simulink model "quadcopterfinal"  (R2015a)
settings: Solver=ode45  SolverMode=SingleTasking  StartTime=0.0  StopTime=10  MaxStep=0.02  RelTol=1e-3
InitFcn:
  | parameters
undefined symbols (not defined in the file or in its folder): kd_roll_rate, kd_yaw_rate, kd_z_rate, ki_roll_rate, ki_yaw_rate, ki_z_rate, kp_roll, kp_roll_rate, kp_yaw, kp_yaw_rate, kp_z, kp_z_rate
libraries: simulink x4
settings Model: CovMetricSettings=dwe  CovHtmlReporting=off  covSaveCumulativeToWorkspaceVar=off  CovSaveSingleToWorkspaceVar=off  CovExternalEMLEnable=on  Creator=manoj  LastModifiedBy=manoj
settings DataIOCC: LimitDataPoints=off  SaveFormat=Dataset
settings DebuggingCC: SFUnexpectedBacktrackingDiag=error  SFNoUnconditionalDefaultTransitionDiag=error
settings HardwareCC: ProdBitPerPointer=64  ProdLargestAtomicFloat=Float  ProdIntDivRoundTo=Zero  ProdEndianess=LittleEndian  ProdHWDeviceType=Specified
settings ModelReferenceCC: PropagateSignalLabelsOutOfModel=on
settings GRTTargetCC: TargetLangStandard=C99 (ISO)  GeneratePreprocessorConditionals=Use local settings

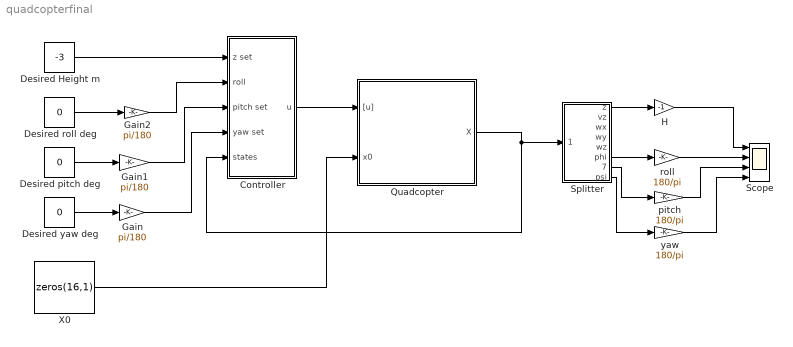
== system quadcopterfinal ==
  Controller : Subsystem
  Desired Height m : Constant  Value=-3
  Desired pitch deg : Constant  Value=0
  Desired roll deg : Constant  Value=0
  Desired yaw deg : Constant  Value=0
  Gain : Gain  Gain=pi/180
  Gain1 : Gain  Gain=pi/180
  Gain2 : Gain  Gain=pi/180
  H : Gain  Gain=-1
  Quadcopter : Subsystem
      mask Display: image('/home/manoj/gits/DDP_work/FCB related/quadcopter simulation/quad render 1(1).png');
  Scope : Scope  NumInputPorts=4
      settings: TimeRange=auto  ShowLegends=on  MaxDataPoints=5000  SaveToWorkspace=off  SaveName=ScopeData  YMin=-551.8125~-5~-5~-5  YMax=61.3125~5~5~5  SampleTime=-1
  Splitter : MATLAB Function  TreatAsAtomicUnit=on
      settings: PermitHierarchicalResolution=ParametersOnly
  X0 : Constant  Value=zeros(16,1)
  pitch : Gain  Gain=180/pi
  roll : Gain  Gain=180/pi
  yaw : Gain  Gain=180/pi
  wires:
  X0/1 -> Quadcopter/2(x0)
  Quadcopter/1(X) -> Splitter/1(states), Controller/5(states)
  Desired Height m/1 -> Controller/1(z set)
  Desired roll deg/1 -> Gain2/1
  Desired pitch deg/1 -> Gain1/1
  Desired yaw deg/1 -> Gain/1
  Controller/1(u) -> Quadcopter/1("[u]")
  Splitter/1(z) -> H/1
  Splitter/7(theta) -> pitch/1
  Splitter/8(psi) -> yaw/1
  H/1 -> Scope/1
  Gain1/1 -> Controller/3(pitch set)
  Gain/1 -> Controller/4(yaw set)
  roll/1 -> Scope/2
  pitch/1 -> Scope/3
  yaw/1 -> Scope/4
  Splitter/6(phi) -> roll/1
  Gain2/1 -> Controller/2(roll)

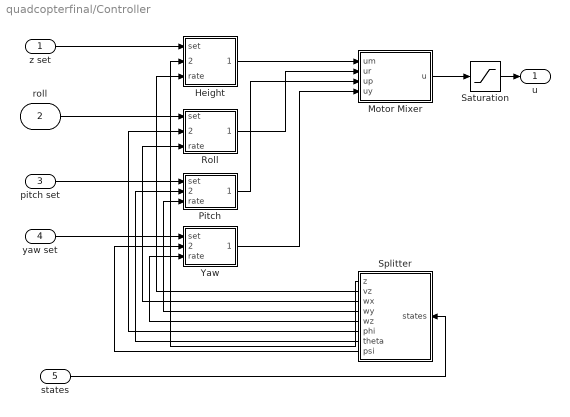
== system quadcopterfinal/Controller ==
  z set : Inport
  roll : Inport  Port=2
  pitch set : Inport  Port=3
  yaw set : Inport  Port=4
  states : Inport  Port=5
  Height : Subsystem
  Motor Mixer : MATLAB Function  TreatAsAtomicUnit=on
      settings: PermitHierarchicalResolution=ParametersOnly
  Pitch : Subsystem
  Roll : Subsystem
  Saturation : Saturate  UpperLimit=1  LowerLimit=0
  Splitter : MATLAB Function  TreatAsAtomicUnit=on
      settings: PermitHierarchicalResolution=ParametersOnly
  Yaw : Subsystem
  u : Outport
  wires:
  Splitter/3(wx) -> Roll/3(rate)
  Splitter/7(theta) -> Pitch/2(state)
  Splitter/1(z) -> Height/2(state)
  Splitter/8(psi) -> Yaw/2(state)
  Motor Mixer/1(u) -> Saturation/1
  z set/1 -> Height/1(set)
  Height/1(Out1) -> Motor Mixer/1(um)
  Roll/1(Out1) -> Motor Mixer/2(ur)
  Pitch/1(Out1) -> Motor Mixer/3(up)
  Yaw/1(Out1) -> Motor Mixer/4(uy)
  roll/1 -> Roll/1(set)
  pitch set/1 -> Pitch/1(set)
  yaw set/1 -> Yaw/1(set)
  Splitter/4(wy) -> Pitch/3(rate)
  Splitter/2(vz) -> Height/3(rate)
  Splitter/6(phi) -> Roll/2(state)
  Splitter/5(wz) -> Yaw/3(rate)
  Saturation/1 -> u/1
  states/1 -> Splitter/1(states)

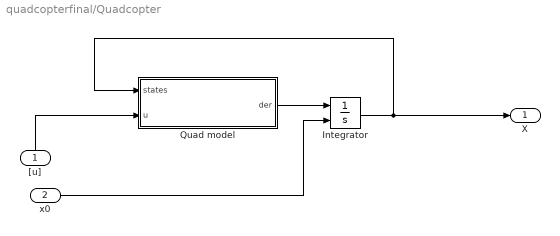
== system quadcopterfinal/Quadcopter ==
  "[u]" : Inport
  x0 : Inport  Port=2
  Integrator : Integrator  InitialConditionSource=external  LimitOutput=on  UpperSaturationLimit=[inf,inf,inf,inf,inf,inf,inf,inf,inf,inf,inf,inf,inf,inf,inf,inf]'  LowerSaturationLimit=-[inf,inf,inf,inf,inf,inf,inf,inf,inf,inf,inf,inf,0,0,0,0]'
  Quad model : MATLAB Function  TreatAsAtomicUnit=on
      settings: PermitHierarchicalResolution=ParametersOnly
  X : Outport
  wires:
  x0/1 -> Integrator/2
  Quad model/1(der) -> Integrator/1
  "[u]"/1 -> Quad model/2(u)
  Integrator/1 -> X/1, Quad model/1(states)

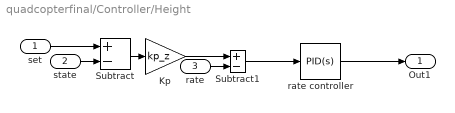
== system quadcopterfinal/Controller/Height ==
  set : Inport
  state : Inport  Port=2
  rate : Inport  Port=3
  Kp : Gain  Gain=kp_z
  Subtract : Sum  Inputs=+-
  Subtract1 : Sum  Inputs=+-
  rate controller : simulink/Continuous/PID Controller  Controller=PID  TimeDomain=Continuous-time  SampleTime=-1  IntegratorMethod=Forward Euler  FilterMethod=Forward Euler  Form=Parallel  UseFilter=on  ControllerParametersSource=internal  P=kp_z_rate  I=ki_z_rate  D=kd_z_rate  N=10  InitialConditionSource=internal  InitialConditionForIntegrator=0  InitialConditionForFilter=0  ExternalReset=none  LimitOutput=on  UpperSaturationLimit=0.5  LowerSaturationLimit=-0.5  LinearizeAsGain=on  AntiWindupMode=clamping  Kb=1  TrackingMode=off  Kt=1  PParamMin=[]  PParamMax=[]  IParamMin=[]  IParamMax=[]  DParamMin=[]  DParamMax=[]  NParamMin=[]  NParamMax=[]  KbParamMin=[]  KbParamMax=[]  KtParamMin=[]  KtParamMax=[]  POutMin=[]  POutMax=[]  IOutMin=[]  IOutMax=[]  DOutMin=[]  DOutMax=[]  NOutMin=[]  NOutMax=[]  KbOutMin=[]  KbOutMax=[]  KtOutMin=[]  KtOutMax=[]  IntegratorOutMin=[]  IntegratorOutMax=[]  FilterOutMin=[]  FilterOutMax=[]  SumOutMin=[]  SumOutMax=[]  SumI1OutMin=[]  SumI1OutMax=[]  SumI2OutMin=[]  SumI2OutMax=[]  SumI3OutMin=[]  SumI3OutMax=[]  SumDOutMin=[]  SumDOutMax=[]  SaturationOutMin=[]  SaturationOutMax=[]  IntegratorContinuousStateAttributes=''  IntegratorStateMustResolveToSignalObject=off  IntegratorRTWStateStorageClass=Auto  FilterContinuousStateAttributes=''  FilterStateMustResolveToSignalObject=off  FilterRTWStateStorageClass=Auto  DifferentiatorICPrevScaledInput=0  DifferentiatorOutMin=[]  DifferentiatorOutMax=[]
  Out1 : Outport
  wires:
  Subtract/1 -> Kp/1
  Subtract1/1 -> rate controller/1
  state/1 -> Subtract/2
  Kp/1 -> Subtract1/1
  set/1 -> Subtract/1
  rate/1 -> Subtract1/2
  rate controller/1 -> Out1/1

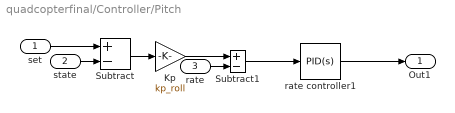
== system quadcopterfinal/Controller/Pitch ==
  set : Inport
  state : Inport  Port=2
  rate : Inport  Port=3
  Kp : Gain  Gain=kp_roll
  Subtract : Sum  Inputs=+-
  Subtract1 : Sum  Inputs=+-
  rate controller1 : simulink/Continuous/PID Controller  Controller=PID  TimeDomain=Continuous-time  SampleTime=-1  IntegratorMethod=Forward Euler  FilterMethod=Forward Euler  Form=Parallel  UseFilter=on  ControllerParametersSource=internal  P=kp_roll_rate  I=ki_roll_rate  D=kd_roll_rate  N=10  InitialConditionSource=internal  InitialConditionForIntegrator=0  InitialConditionForFilter=0  ExternalReset=none  LimitOutput=on  UpperSaturationLimit=00.5  LowerSaturationLimit=-0.5  LinearizeAsGain=on  AntiWindupMode=clamping  Kb=1  TrackingMode=off  Kt=1  PParamMin=[]  PParamMax=[]  IParamMin=[]  IParamMax=[]  DParamMin=[]  DParamMax=[]  NParamMin=[]  NParamMax=[]  KbParamMin=[]  KbParamMax=[]  KtParamMin=[]  KtParamMax=[]  POutMin=[]  POutMax=[]  IOutMin=[]  IOutMax=[]  DOutMin=[]  DOutMax=[]  NOutMin=[]  NOutMax=[]  KbOutMin=[]  KbOutMax=[]  KtOutMin=[]  KtOutMax=[]  IntegratorOutMin=[]  IntegratorOutMax=[]  FilterOutMin=[]  FilterOutMax=[]  SumOutMin=[]  SumOutMax=[]  SumI1OutMin=[]  SumI1OutMax=[]  SumI2OutMin=[]  SumI2OutMax=[]  SumI3OutMin=[]  SumI3OutMax=[]  SumDOutMin=[]  SumDOutMax=[]  SaturationOutMin=[]  SaturationOutMax=[]  IntegratorContinuousStateAttributes=''  IntegratorStateMustResolveToSignalObject=off  IntegratorRTWStateStorageClass=Auto  FilterContinuousStateAttributes=''  FilterStateMustResolveToSignalObject=off  FilterRTWStateStorageClass=Auto  DifferentiatorICPrevScaledInput=0  DifferentiatorOutMin=[]  DifferentiatorOutMax=[]
  Out1 : Outport
  wires:
  Subtract/1 -> Kp/1
  Subtract1/1 -> rate controller1/1
  state/1 -> Subtract/2
  Kp/1 -> Subtract1/1
  set/1 -> Subtract/1
  rate/1 -> Subtract1/2
  rate controller1/1 -> Out1/1

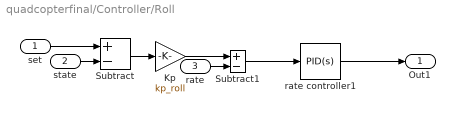
== system quadcopterfinal/Controller/Roll ==
  set : Inport
  state : Inport  Port=2
  rate : Inport  Port=3
  Kp : Gain  Gain=kp_roll
  Subtract : Sum  Inputs=+-
  Subtract1 : Sum  Inputs=+-
  rate controller1 : simulink/Continuous/PID Controller  Controller=PID  TimeDomain=Continuous-time  SampleTime=-1  IntegratorMethod=Forward Euler  FilterMethod=Forward Euler  Form=Parallel  UseFilter=on  ControllerParametersSource=internal  P=kp_roll_rate  I=ki_roll_rate  D=kd_roll_rate  N=10  InitialConditionSource=internal  InitialConditionForIntegrator=0  InitialConditionForFilter=0  ExternalReset=none  LimitOutput=on  UpperSaturationLimit=0.5  LowerSaturationLimit=-0.5  LinearizeAsGain=on  AntiWindupMode=clamping  Kb=1  TrackingMode=off  Kt=1  PParamMin=[]  PParamMax=[]  IParamMin=[]  IParamMax=[]  DParamMin=[]  DParamMax=[]  NParamMin=[]  NParamMax=[]  KbParamMin=[]  KbParamMax=[]  KtParamMin=[]  KtParamMax=[]  POutMin=[]  POutMax=[]  IOutMin=[]  IOutMax=[]  DOutMin=[]  DOutMax=[]  NOutMin=[]  NOutMax=[]  KbOutMin=[]  KbOutMax=[]  KtOutMin=[]  KtOutMax=[]  IntegratorOutMin=[]  IntegratorOutMax=[]  FilterOutMin=[]  FilterOutMax=[]  SumOutMin=[]  SumOutMax=[]  SumI1OutMin=[]  SumI1OutMax=[]  SumI2OutMin=[]  SumI2OutMax=[]  SumI3OutMin=[]  SumI3OutMax=[]  SumDOutMin=[]  SumDOutMax=[]  SaturationOutMin=[]  SaturationOutMax=[]  IntegratorContinuousStateAttributes=''  IntegratorStateMustResolveToSignalObject=off  IntegratorRTWStateStorageClass=Auto  FilterContinuousStateAttributes=''  FilterStateMustResolveToSignalObject=off  FilterRTWStateStorageClass=Auto  DifferentiatorICPrevScaledInput=0  DifferentiatorOutMin=[]  DifferentiatorOutMax=[]
  Out1 : Outport
  wires:
  Subtract/1 -> Kp/1
  Subtract1/1 -> rate controller1/1
  state/1 -> Subtract/2
  Kp/1 -> Subtract1/1
  set/1 -> Subtract/1
  rate/1 -> Subtract1/2
  rate controller1/1 -> Out1/1

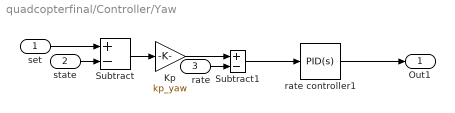
== system quadcopterfinal/Controller/Yaw ==
  set : Inport
  state : Inport  Port=2
  rate : Inport  Port=3
  Kp : Gain  Gain=kp_yaw
  Subtract : Sum  Inputs=+-
  Subtract1 : Sum  Inputs=+-
  rate controller1 : simulink/Continuous/PID Controller  Controller=PID  TimeDomain=Continuous-time  SampleTime=-1  IntegratorMethod=Forward Euler  FilterMethod=Forward Euler  Form=Parallel  UseFilter=on  ControllerParametersSource=internal  P=kp_yaw_rate  I=ki_yaw_rate  D=kd_yaw_rate  N=10  InitialConditionSource=internal  InitialConditionForIntegrator=0  InitialConditionForFilter=0  ExternalReset=none  LimitOutput=on  UpperSaturationLimit=0.5  LowerSaturationLimit=-0.5  LinearizeAsGain=on  AntiWindupMode=clamping  Kb=1  TrackingMode=off  Kt=1  PParamMin=[]  PParamMax=[]  IParamMin=[]  IParamMax=[]  DParamMin=[]  DParamMax=[]  NParamMin=[]  NParamMax=[]  KbParamMin=[]  KbParamMax=[]  KtParamMin=[]  KtParamMax=[]  POutMin=[]  POutMax=[]  IOutMin=[]  IOutMax=[]  DOutMin=[]  DOutMax=[]  NOutMin=[]  NOutMax=[]  KbOutMin=[]  KbOutMax=[]  KtOutMin=[]  KtOutMax=[]  IntegratorOutMin=[]  IntegratorOutMax=[]  FilterOutMin=[]  FilterOutMax=[]  SumOutMin=[]  SumOutMax=[]  SumI1OutMin=[]  SumI1OutMax=[]  SumI2OutMin=[]  SumI2OutMax=[]  SumI3OutMin=[]  SumI3OutMax=[]  SumDOutMin=[]  SumDOutMax=[]  SaturationOutMin=[]  SaturationOutMax=[]  IntegratorContinuousStateAttributes=''  IntegratorStateMustResolveToSignalObject=off  IntegratorRTWStateStorageClass=Auto  FilterContinuousStateAttributes=''  FilterStateMustResolveToSignalObject=off  FilterRTWStateStorageClass=Auto  DifferentiatorICPrevScaledInput=0  DifferentiatorOutMin=[]  DifferentiatorOutMax=[]
  Out1 : Outport
  wires:
  Subtract/1 -> Kp/1
  Subtract1/1 -> rate controller1/1
  state/1 -> Subtract/2
  Kp/1 -> Subtract1/1
  set/1 -> Subtract/1
  rate/1 -> Subtract1/2
  rate controller1/1 -> Out1/1

== matlab function quadcopterfinal/Controller/Motor Mixer ==
  data: um input; u output; ur input; up input; uy input
function u = fcn(um, ur, up, uy)
 u = zeros(4,1);
 um = 0.4+um;
  u(1) = um + up -ur + uy;
  u(2) = um - up +ur + uy;
  u(3) = um + up +ur - uy;
  u(4) = um - up -ur - uy;
  u = -u;

== matlab function quadcopterfinal/Quadcopter/Quad model ==
  data: states input; u input; der output
function der   = Quadcopter_nonLinear( states , u )
%returns the derivative of the current states based on Quadcopters
%mathematical model. der stands for derivative
%SI units unless specified for all the states and params
x = states(1);
y = states(2);
z = states(3);
vx = states(4);
vy = states(5);
vz = states(6);
wx =states(7);
wy = states(8);
wz = states(9);
psi = states(10); 
theta = states(11);
phi = states(12);
w = states(13:16);

%% Constants
%8x4.5 propeller. 850kv Avionic our standard motor choice. 
A = 2.1098e-07 ; %motor propeller related constants
B = 2.9350e+03 ; %motor propeller related constants
C = 0.0030     ; %motor propeller related constants
D = 5.29*10^-6     ; %Thrust constant
E = 0.063*10^-6    ; %ktau of prop
L = 0.25;       %half of diagonal
Mass = 0.9;
Iquad = [0.0180  0      0 
            0   0.018   0
            0     0   0.026];
g = 9.81;
%% Thrust and Moments
T = D * w.^2;
totalThrust = sum(T);
Mx = (-T(1) + T(2) + T(3) - T(4))*L*E/D/sqrt(2);
My = (+T(1) - T(2) + T(3) - T(4))*L*E/D/sqrt(2);
Mz = (+T(1) + T(2) - T(3) - T(4))*L*E/D/sqrt(2);

%% Model
%Rotation Matrix
c_psi = cos(psi);
s_psi = sin(psi);
c_theta = cos(theta);
s_theta = sin(theta);
c_phi = cos(phi);
s_phi = sin(phi);
Cy = [c_psi  , s_psi  , 0;
      -s_psi , c_psi  , 0; 
      0      ,   0    , 1];
Cp = [c_theta    , 0 , -s_theta;
        0        , 1 ,    0   ;
     s_theta     , 0 , c_theta];
Cr = [1 ,      0        ,  0;
      0 ,   c_phi       , s_phi;
      0 ,   -s_phi      , c_phi];
Cbi = Cr*Cp*Cy;

%converting body rates to euler rates
rpy_dot = [1, s_theta/c_theta*s_phi, s_theta/c_theta*c_phi;
           0, c_phi                , -s_phi;
           0, s_phi/c_phi          , c_phi/c_theta         ] * [wx; wy; wz]; 
der = zeros(16,1);
der(1:3) = [vx; vy; vz];
%Cbi mat is rotation matrix. RM' =inv(RM)
der(4:6) = [0; 0; g] + (Cbi')*[0; 0; -totalThrust/Mass];
der(7:9) = [Mx/Iquad(1,1); My/Iquad(2,2); Mz/Iquad(3,3)] + ...
            [(Iquad(2,2) - Iquad(3,3) )/ Iquad(1,1)*wy*wz;
             (Iquad(3,3) - Iquad(1,1) )/ Iquad(2,2)*wx*wz;
             (Iquad(1,1) - Iquad(2,2) )/ Iquad(3,3)*wx*wy;];
der(10:12) = [rpy_dot(3); rpy_dot(2); rpy_dot(1)];
der(13:16) = B * u - A * w - C * w.*w;          

end

== matlab function quadcopterfinal/Controller/Splitter ==
  data: states input; z output; vz output; wx output; wy output; wz output; phi output; theta output; psi output
function [z,vz,wx,wy,wz,phi,theta,psi] = fcn(states)
x = states(1);
y = states(2);
z = states(3);
vx = states(4);
vy = states(5);
vz = states(6);
wx =states(7);
wy = states(8);
wz = states(9);
psi = states(10); 
theta = states(11);
phi = states(12);
w = states(13:16);

== matlab function quadcopterfinal/Splitter ==
  data: states input; z output; vz output; wx output; wy output; wz output; phi output; theta output; psi output
function [z,vz,wx,wy,wz,phi,theta,psi] = fcn(states)
x = states(1);
y = states(2);
z = states(3);
vx = states(4);
vy = states(5);
vz = states(6);
wx =states(7);
wy = states(8);
wz = states(9);
psi = states(10); 
theta = states(11);
phi = states(12);
w = states(13:16);
